simulink model "MIMOOO_FIXED"  (R2022a)
settings: Solver=VariableStepAuto  StartTime=0.0  StopTime=100  RelTol=1e-3
libraries: dspsigops x80, commchan3 x4, commdigbbndpm3 x2, commfilt2 x2, commsink2 x1, simulink x1
(part 4 of 6)

== system MIMOOO_FIXED/Transceiver1/Interpolation 2/E7 ==
  In1 : Inport
  Data Type Conversion1 : DataTypeConversion  OutDataTypeStr=fixdt(1,19,0)  RndMeth=Floor
  Data Type Conversion12 : DataTypeConversion  OutDataTypeStr=fixdt(1,17,0)  RndMeth=Floor
  Data Type Conversion2 : DataTypeConversion  OutDataTypeStr=fixdt(1,18,0)  RndMeth=Floor
  Data Type Conversion3 : DataTypeConversion  OutDataTypeStr=fixdt(1,19,0)  RndMeth=Floor
  Delay6 : Delay  DelayLength=1
  Delay7 : Delay  DelayLength=1
  Gain4 : Gain  Gain=56
  Gain5 : Gain  Gain=336
  Gain6 : Gain  Gain=120
  Sum4 : Sum
  Sum5 : Sum
  Out1 : Outport
  wires:
  Gain4/1 -> Data Type Conversion12/1
  Sum4/1 -> Data Type Conversion3/1
  Delay7/1 -> Sum5/2
  Gain6/1 -> Data Type Conversion2/1
  Delay6/1 -> Sum4/2
  Data Type Conversion12/1 -> Delay6/1
  Gain5/1 -> Data Type Conversion1/1
  Data Type Conversion1/1 -> Sum4/1
  Data Type Conversion2/1 -> Sum5/1
  Data Type Conversion3/1 -> Delay7/1
  In1/1 -> Gain6/1, Gain5/1, Gain4/1
  Sum5/1 -> Out1/1

== system MIMOOO_FIXED/Transceiver5/ADC 1/SigmaDelta ADC ==
  note: c1
  In : Inport
  Discrete Transfer Fcn : DiscreteTransferFcn  Denominator=[1 -1]
  Discrete Transfer Fcn1 : DiscreteTransferFcn  Numerator=[1 0]  Denominator=[1 -1]
  Discrete Transfer Fcn2 : DiscreteTransferFcn  Denominator=[1 -1]
  Discrete Transfer Fcn3 : DiscreteTransferFcn  Numerator=[1 0]  Denominator=[1 -1]
  Discrete Transfer Fcn4 : DiscreteTransferFcn  Denominator=[1 -1]
  Discrete Transfer Fcn5 : DiscreteTransferFcn  Numerator=[1 0]  Denominator=[1 -1]
  Sign : Signum
  Sum : Sum  Inputs=-++  InputSameDT=on  SaturateOnIntegerOverflow=on  OutDataTypeStr=Inherit: Same as first input
  Sum1 : Sum  Inputs=-+  InputSameDT=on  SaturateOnIntegerOverflow=on  OutDataTypeStr=Inherit: Same as first input
  Sum3 : Sum  Inputs=-+  InputSameDT=on  SaturateOnIntegerOverflow=on  OutDataTypeStr=Inherit: Same as first input
  Sum4 : Sum  Inputs=++++++  InputSameDT=on  SaturateOnIntegerOverflow=on  OutDataTypeStr=Inherit: Same as first input
  a : Gain  Gain=-1  SaturateOnIntegerOverflow=on  OutDataTypeStr=Inherit: Same as input  ParamDataTypeStr=Inherit: Same as input
  a1 : Gain  Gain=0.556869897897495  SaturateOnIntegerOverflow=on  OutDataTypeStr=Inherit: Same as input  ParamDataTypeStr=Inherit: Same as input
  a2 : Gain  Gain=-0.556869897925717  SaturateOnIntegerOverflow=on  OutDataTypeStr=Inherit: Same as input  ParamDataTypeStr=Inherit: Same as input
  a3 : Gain  Gain=5.57074843011795e-10  SaturateOnIntegerOverflow=on  OutDataTypeStr=Inherit: Same as input  ParamDataTypeStr=Inherit: Same as input
  a4 : Gain  Gain=-0.239860502762260  SaturateOnIntegerOverflow=on  OutDataTypeStr=Inherit: Same as input  ParamDataTypeStr=Inherit: Same as input
  a5 : Gain  Gain=-0.0411685762497780  SaturateOnIntegerOverflow=on  OutDataTypeStr=Inherit: Same as input  ParamDataTypeStr=Inherit: Same as input
  a6 : Gain  Gain=0.0229325751731016  SaturateOnIntegerOverflow=on  OutDataTypeStr=Inherit: Same as input  ParamDataTypeStr=Inherit: Same as input
  gc1 : Gain  Gain=2.00000000000000  SaturateOnIntegerOverflow=on  OutDataTypeStr=Inherit: Same as input  ParamDataTypeStr=Inherit: Same as input
  gc2 : Gain  Gain=2.07602752770857  SaturateOnIntegerOverflow=on  OutDataTypeStr=Inherit: Same as input  ParamDataTypeStr=Inherit: Same as input
  gc3 : Gain  Gain=1.92397247229143  SaturateOnIntegerOverflow=on  OutDataTypeStr=Inherit: Same as input  ParamDataTypeStr=Inherit: Same as input
  Out : Outport
  wires:
  gc1/1 -> Sum/1
  a5/1 -> Sum4/2
  Discrete Transfer Fcn2/1 -> Discrete Transfer Fcn3/1, a3/1
  Sum4/1 -> Sign/1
  Sum1/1 -> Discrete Transfer Fcn2/1
  Sum/1 -> Discrete Transfer Fcn/1
  a1/1 -> Sum4/6
  gc2/1 -> Sum1/1
  a/1 -> Sum/3
  Discrete Transfer Fcn3/1 -> a4/1, Sum3/2, gc2/1
  Discrete Transfer Fcn5/1 -> a6/1, gc3/1
  Discrete Transfer Fcn1/1 -> a2/1, gc1/1, Sum1/2
  In/1 -> Sum/2
  Sign/1 -> Out/1, a/1
  gc3/1 -> Sum3/1
  a3/1 -> Sum4/4
  a4/1 -> Sum4/3
  a2/1 -> Sum4/5
  Discrete Transfer Fcn/1 -> Discrete Transfer Fcn1/1, a1/1
  Sum3/1 -> Discrete Transfer Fcn4/1
  Discrete Transfer Fcn4/1 -> Discrete Transfer Fcn5/1, a5/1
  a6/1 -> Sum4/1

== system MIMOOO_FIXED/Transceiver5/Interpolation 1/Half_band ==
  Input : Inport
  Add2 : Sum
  Delay11 : Delay  DelayLength=1
  E0(Z) : Subsystem
  E1(Z) : Subsystem
  Upsample 1 : dspsigops/Upsample  N=2  phase=0  RateOptions=Allow multirate processing  ic=0  mode=Unused parameter value
  Upsample 2 : dspsigops/Upsample  N=2  phase=0  RateOptions=Allow multirate processing  ic=0  mode=Unused parameter value
  Out1 : Outport
  wires:
  Upsample 2/1 -> Delay11/1
  Upsample 1/1 -> Add2/1
  E1(Z)/1(Output) -> Upsample 2/1
  Delay11/1 -> Add2/2
  E0(Z)/1(Out1) -> Upsample 1/1
  Add2/1 -> Out1/1
  Input/1 -> E0(Z)/1(Input), E1(Z)/1(Input1)

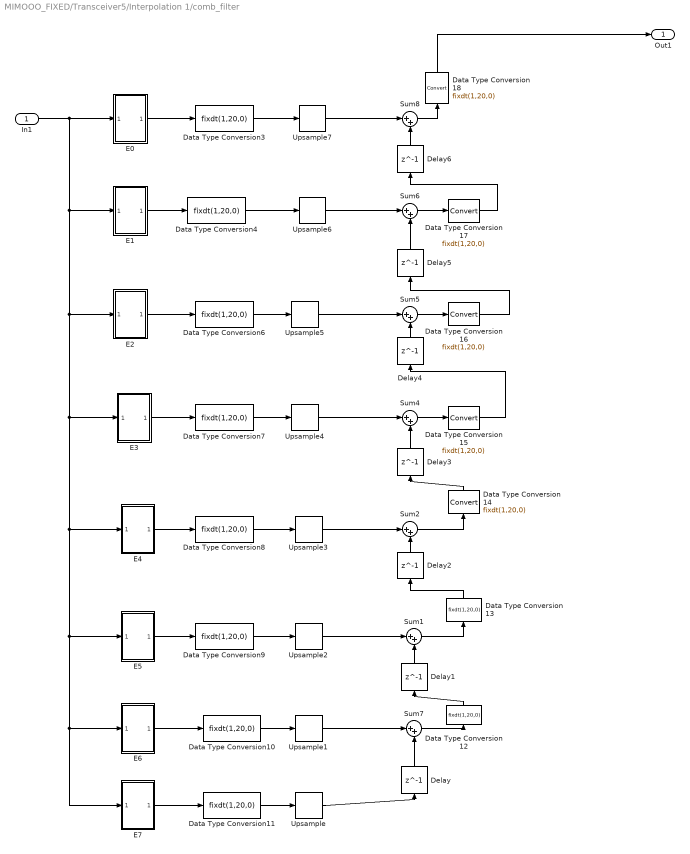
== system MIMOOO_FIXED/Transceiver5/Interpolation 1/comb_filter ==
  In1 : Inport
  Data Type Conversion{3..4,6..18} (15 alike) : DataTypeConversion  OutDataTypeStr=fixdt(1,20,0)  RndMeth=Floor
  Delay{,1..6} (7 alike) : Delay  DelayLength=1
  E0 : Subsystem
  E1 : Subsystem
  E2 : Subsystem
  E3 : Subsystem
  E4 : Subsystem
  E5 : Subsystem
  E6 : Subsystem
  E7 : Subsystem
  Sum{1..2,4..8} (7 alike) : Sum  Inputs=|++
  Upsample{,1..7} (8 alike) : dspsigops/Upsample  N=8  phase=0  RateOptions=Allow multirate processing  ic=0  mode=Unused parameter value
  Out1 : Outport
  wires:
  Upsample7/1 -> Sum8/1
  E4/1(Out1) -> Data Type Conversion8/1
  Data Type Conversion4/1 -> Upsample6/1
  E6/1(Out1) -> Data Type Conversion10/1
  Delay4/1 -> Sum5/2
  Data Type Conversion13/1 -> Delay2/1
  Delay5/1 -> Sum6/2
  Data Type Conversion9/1 -> Upsample2/1
  Sum8/1 -> Data Type Conversion18/1
  Data Type Conversion3/1 -> Upsample7/1
  Sum6/1 -> Data Type Conversion17/1
  Data Type Conversion15/1 -> Delay4/1
  Data Type Conversion14/1 -> Delay3/1
  Data Type Conversion16/1 -> Delay5/1
  E2/1(Out1) -> Data Type Conversion6/1
  In1/1 -> E0/1(In1), E7/1(In1), E6/1(In1), E5/1(In1), E4/1(In1), E3/1(In1), E2/1(In1), E1/1(In1)
  Delay2/1 -> Sum2/2
  Data Type Conversion17/1 -> Delay6/1
  Sum7/1 -> Data Type Conversion12/1
  Data Type Conversion6/1 -> Upsample5/1
  Sum2/1 -> Data Type Conversion14/1
  Data Type Conversion10/1 -> Upsample1/1
  Upsample/1 -> Delay/1
  Upsample6/1 -> Sum6/1
  E5/1(Out1) -> Data Type Conversion9/1
  Data Type Conversion8/1 -> Upsample3/1
  Data Type Conversion7/1 -> Upsample4/1
  Delay1/1 -> Sum1/2
  Sum5/1 -> Data Type Conversion16/1
  Delay/1 -> Sum7/2
  Upsample3/1 -> Sum2/1
  Data Type Conversion11/1 -> Upsample/1
  Upsample4/1 -> Sum4/1
  E7/1(Out1) -> Data Type Conversion11/1
  Sum1/1 -> Data Type Conversion13/1
  Delay3/1 -> Sum4/2
  E3/1(Out1) -> Data Type Conversion7/1
  Data Type Conversion12/1 -> Delay1/1
  Sum4/1 -> Data Type Conversion15/1
  Upsample2/1 -> Sum1/1
  Upsample5/1 -> Sum5/1
  Upsample1/1 -> Sum7/1
  E1/1(Out1) -> Data Type Conversion4/1
  Delay6/1 -> Sum8/2
  Data Type Conversion18/1 -> Out1/1
  E0/1(Out1) -> Data Type Conversion3/1

== system MIMOOO_FIXED/Transceiver5/Interpolation 2/E0 ==
  In1 : Inport
  Data Type Conversion1 : DataTypeConversion  OutDataTypeStr=fixdt(1,19,0)  RndMeth=Floor
  Data Type Conversion2 : DataTypeConversion  OutDataTypeStr=fixdt(1,18,0)  RndMeth=Floor
  Data Type Conversion3 : DataTypeConversion  OutDataTypeStr=fixdt(1,11,0)  RndMeth=Floor
  Data Type Conversion4 : DataTypeConversion  OutDataTypeStr=fixdt(1,20,0)  RndMeth=Floor
  Data Type Conversion5 : DataTypeConversion  OutDataTypeStr=fixdt(1,20,0)  RndMeth=Floor
  Data Type Conversion7 : DataTypeConversion  OutDataTypeStr=fixdt(1,16,0)  RndMeth=Floor
  Delay3 : Delay  DelayLength=1
  Delay4 : Delay  DelayLength=1
  Delay5 : Delay  DelayLength=1
  Gain : Gain  Gain=35
  Gain1 : Gain  Gain=315
  Gain2 : Gain  Gain=161
  Gain3 : Gain
  Sum : Sum
  Sum1 : Sum
  Sum2 : Sum
  Out1 : Outport
  wires:
  Sum1/1 -> Data Type Conversion5/1
  Delay3/1 -> Sum/2
  Delay5/1 -> Sum2/2
  Data Type Conversion7/1 -> Delay3/1
  Gain/1 -> Data Type Conversion7/1
  Gain1/1 -> Data Type Conversion1/1
  Data Type Conversion1/1 -> Sum/1
  Gain2/1 -> Data Type Conversion2/1
  Data Type Conversion3/1 -> Sum2/1
  Gain3/1 -> Data Type Conversion3/1
  Sum/1 -> Data Type Conversion4/1
  Data Type Conversion4/1 -> Delay4/1
  Data Type Conversion2/1 -> Sum1/1
  Delay4/1 -> Sum1/2
  Data Type Conversion5/1 -> Delay5/1
  In1/1 -> Gain2/1, Gain3/1, Gain1/1, Gain/1
  Sum2/1 -> Out1/1

== system MIMOOO_FIXED/Transceiver5/Interpolation 2/E0(Z) ==
  Input : Inport
  Data Type Conversion5 : DataTypeConversion  OutDataTypeStr=fixdt(1,23,0)  RndMeth=Floor
  Delay : Delay  DelayLength=5
  Gain : Gain  Gain=256
  Out1 : Outport
  wires:
  Input/1 -> Gain/1
  Delay/1 -> Out1/1
  Gain/1 -> Data Type Conversion5/1
  Data Type Conversion5/1 -> Delay/1

== system MIMOOO_FIXED/Transceiver5/Interpolation 2/E1 ==
  In1 : Inport
  Data Type Conversion1 : DataTypeConversion  OutDataTypeStr=fixdt(1,19,0)  RndMeth=Floor
  Data Type Conversion2 : DataTypeConversion  OutDataTypeStr=fixdt(1,19,0)  RndMeth=Floor
  Data Type Conversion3 : DataTypeConversion  OutDataTypeStr=fixdt(1,13,0)  RndMeth=Floor
  Data Type Conversion4 : DataTypeConversion  OutDataTypeStr=fixdt(1,19,0)  RndMeth=Floor
  Data Type Conversion5 : DataTypeConversion  OutDataTypeStr=fixdt(1,20,0)  RndMeth=Floor
  Data Type Conversion7 : DataTypeConversion  OutDataTypeStr=fixdt(1,15,0)  RndMeth=Floor
  Delay3 : Delay  DelayLength=1
  Delay4 : Delay  DelayLength=1
  Delay5 : Delay  DelayLength=1
  Gain : Gain  Gain=20
  Gain1 : Gain  Gain=284
  Gain2 : Gain  Gain=204
  Gain3 : Gain  Gain=4
  Sum : Sum
  Sum1 : Sum
  Sum2 : Sum
  Out1 : Outport
  wires:
  Sum/1 -> Data Type Conversion4/1
  Delay3/1 -> Sum/2
  Delay4/1 -> Sum1/2
  Delay5/1 -> Sum2/2
  Gain/1 -> Data Type Conversion7/1
  Data Type Conversion7/1 -> Delay3/1
  Gain1/1 -> Data Type Conversion1/1
  Data Type Conversion1/1 -> Sum/1
  Gain2/1 -> Data Type Conversion2/1
  Data Type Conversion2/1 -> Sum1/1
  Gain3/1 -> Data Type Conversion3/1
  Data Type Conversion3/1 -> Sum2/1
  Data Type Conversion4/1 -> Delay4/1
  Sum1/1 -> Data Type Conversion5/1
  Data Type Conversion5/1 -> Delay5/1
  In1/1 -> Gain2/1, Gain3/1, Gain1/1, Gain/1
  Sum2/1 -> Out1/1

== system MIMOOO_FIXED/Transceiver5/Interpolation 2/E1(Z) ==
  Input1 : Inport
  10-12 : Gain  Gain=158
  2-20 : Gain
  4-18 : Gain  Gain=-4
  6-16 : Gain  Gain=13
  8-14 : Gain  Gain=-40
  Add{7..10,12..16} (9 alike) : Sum
  Data Type Conversion1 : DataTypeConversion  OutDataTypeStr=fixdt(1,15,0)  RndMeth=Floor
  Data Type Conversion{10..14} (5 alike) : DataTypeConversion  OutDataTypeStr=fixdt(1,23,0)  RndMeth=Floor
  Data Type Conversion2 : DataTypeConversion  OutDataTypeStr=fixdt(1,17,0)  RndMeth=Floor
  Data Type Conversion3 : DataTypeConversion  OutDataTypeStr=fixdt(1,19,0)  RndMeth=Floor
  Data Type Conversion4 : DataTypeConversion  OutDataTypeStr=fixdt(1,20,0)  RndMeth=Floor
  Data Type Conversion5 : DataTypeConversion  OutDataTypeStr=fixdt(1,22,0)  RndMeth=Floor
  Data Type Conversion6 : DataTypeConversion  OutDataTypeStr=fixdt(1,17,0)  RndMeth=Floor
  Data Type Conversion7 : DataTypeConversion  OutDataTypeStr=fixdt(1,19,0)  RndMeth=Floor
  Data Type Conversion8 : DataTypeConversion  OutDataTypeStr=fixdt(1,20,0)  RndMeth=Floor
  Data Type Conversion9 : DataTypeConversion  OutDataTypeStr=fixdt(1,22,0)  RndMeth=Floor
  Delay{21,23,25,27,29,31,33,35,37} (9 alike) : Delay  DelayLength=1
  Output : Outport
  wires:
  8-14/1 -> Data Type Conversion4/1
  Delay29/1 -> Add12/2  "x[n-11]"
  Add14/1 -> Data Type Conversion12/1
  Input1/1 -> 2-20/1, 10-12/1, 8-14/1, 6-16/1, 4-18/1
  4-18/1 -> Data Type Conversion2/1
  Delay33/1 -> Add14/2
  Add12/1 -> Data Type Conversion10/1
  10-12/1 -> Data Type Conversion5/1
  Delay37/1 -> Add16/2  "x[n-19]"
  6-16/1 -> Data Type Conversion3/1
  Delay25/1 -> Add9/2  "x[n-7]"
  Add7/1 -> Data Type Conversion6/1
  Add15/1 -> Data Type Conversion13/1
  Delay23/1 -> Add8/2  "x[n-5]"
  Delay27/1 -> Add10/2  "x[n-9]"
  Delay31/1 -> Add13/2  "x[n-13]"
  Delay35/1 -> Add15/2  "x[n-17]"
  Delay21/1 -> Add7/2  "x[n-3]"
  2-20/1 -> Data Type Conversion1/1
  Add13/1 -> Data Type Conversion11/1
  Add10/1 -> Data Type Conversion9/1
  Data Type Conversion1/1 -> Delay21/1, Add16/1
  Data Type Conversion2/1 -> Add7/1, Add15/1
  Data Type Conversion3/1 -> Add8/1, Add14/1
  Data Type Conversion4/1 -> Add9/1, Add13/1
  Data Type Conversion5/1 -> Add10/1, Add12/1
  Data Type Conversion6/1 -> Delay23/1
  Add8/1 -> Data Type Conversion7/1
  Data Type Conversion7/1 -> Delay25/1
  Add9/1 -> Data Type Conversion8/1
  Data Type Conversion8/1 -> Delay27/1
  Data Type Conversion9/1 -> Delay29/1
  Data Type Conversion10/1 -> Delay31/1
  Data Type Conversion11/1 -> Delay33/1
  Data Type Conversion12/1 -> Delay35/1
  Data Type Conversion13/1 -> Delay37/1
  Add16/1 -> Data Type Conversion14/1
  Data Type Conversion14/1 -> Output/1

== system MIMOOO_FIXED/Transceiver5/Interpolation 2/E2 ==
  In1 : Inport
  Data Type Conversion : DataTypeConversion  OutDataTypeStr=fixdt(1,14,0)  SaturateOnIntegerOverflow=off  RndMeth=Floor
  Data Type Conversion1 : DataTypeConversion  OutDataTypeStr=fixdt(1,19,0)  SaturateOnIntegerOverflow=off  RndMeth=Floor
  Data Type Conversion2 : DataTypeConversion  OutDataTypeStr=fixdt(1,19,0)  SaturateOnIntegerOverflow=off  RndMeth=Floor
  Data Type Conversion3 : DataTypeConversion  OutDataTypeStr=fixdt(1,20,0)  SaturateOnIntegerOverflow=off  RndMeth=Floor
  Delay3 : Delay  DelayLength=1
  Delay4 : Delay  DelayLength=1
  Delay5 : Delay  DelayLength=1
  Gain : Gain  Gain=10
  Gain1 : Gain  Gain=246
  Sum : Sum
  Sum1 : Sum
  Sum2 : Sum
  Out1 : Outport
  wires:
  Sum1/1 -> Data Type Conversion3/1
  Delay3/1 -> Sum/2
  Delay4/1 -> Sum1/2
  Delay5/1 -> Sum2/2
  Data Type Conversion/1 -> Delay3/1, Sum2/1
  Gain/1 -> Data Type Conversion/1
  Gain1/1 -> Data Type Conversion1/1
  Data Type Conversion1/1 -> Sum1/1, Sum/1
  Data Type Conversion2/1 -> Delay4/1
  Sum/1 -> Data Type Conversion2/1
  Data Type Conversion3/1 -> Delay5/1
  In1/1 -> Gain1/1, Gain/1
  Sum2/1 -> Out1/1

== system MIMOOO_FIXED/Transceiver5/Interpolation 2/E3 ==
  In1 : Inport
  Data Type Conversion : DataTypeConversion  OutDataTypeStr=fixdt(1,13,0)  SaturateOnIntegerOverflow=off  RndMeth=Floor
  Data Type Conversion1 : DataTypeConversion  OutDataTypeStr=fixdt(1,19,0)  SaturateOnIntegerOverflow=off  RndMeth=Floor
  Data Type Conversion2 : DataTypeConversion  OutDataTypeStr=fixdt(1,19,0)  SaturateOnIntegerOverflow=off  RndMeth=Floor
  Data Type Conversion3 : DataTypeConversion  OutDataTypeStr=fixdt(1,15,0)  SaturateOnIntegerOverflow=off  RndMeth=Floor
  Data Type Conversion4 : DataTypeConversion  OutDataTypeStr=fixdt(1,19,0)  SaturateOnIntegerOverflow=off  RndMeth=Floor
  Data Type Conversion5 : DataTypeConversion  OutDataTypeStr=fixdt(1,20,0)  SaturateOnIntegerOverflow=off  RndMeth=Floor
  Delay3 : Delay  DelayLength=1
  Delay4 : Delay  DelayLength=1
  Delay5 : Delay  DelayLength=1
  Gain : Gain  Gain=4
  Gain1 : Gain  Gain=204
  Gain2 : Gain  Gain=284
  Gain3 : Gain  Gain=20
  Sum : Sum
  Sum1 : Sum
  Sum2 : Sum
  Out1 : Outport
  wires:
  Delay3/1 -> Sum/2
  Delay4/1 -> Sum1/2
  Delay5/1 -> Sum2/2
  Gain/1 -> Data Type Conversion/1
  Data Type Conversion/1 -> Delay3/1
  Gain1/1 -> Data Type Conversion1/1
  Data Type Conversion1/1 -> Sum/1
  Gain2/1 -> Data Type Conversion2/1
  Data Type Conversion2/1 -> Sum1/1
  Gain3/1 -> Data Type Conversion3/1
  Data Type Conversion3/1 -> Sum2/1
  Sum/1 -> Data Type Conversion4/1
  Data Type Conversion4/1 -> Delay4/1
  Sum1/1 -> Data Type Conversion5/1
  Data Type Conversion5/1 -> Delay5/1
  Sum2/1 -> Out1/1
  In1/1 -> Gain3/1, Gain2/1, Gain1/1, Gain/1

== system MIMOOO_FIXED/Transceiver5/Interpolation 2/E4 ==
  In1 : Inport
  Data Type Conversion1 : DataTypeConversion  OutDataTypeStr=fixdt(1,18,0)  RndMeth=Floor
  Data Type Conversion12 : DataTypeConversion  OutDataTypeStr=fixdt(1,11,0)  RndMeth=Floor
  Data Type Conversion2 : DataTypeConversion  OutDataTypeStr=fixdt(1,19,0)  RndMeth=Floor
  Data Type Conversion3 : DataTypeConversion  OutDataTypeStr=fixdt(1,16,0)  RndMeth=Floor
  Data Type Conversion4 : DataTypeConversion  OutDataTypeStr=fixdt(1,18,0)  RndMeth=Floor
  Data Type Conversion5 : DataTypeConversion  OutDataTypeStr=fixdt(1,19,0)  RndMeth=Floor
  Delay3 : Delay  DelayLength=1
  Delay4 : Delay  DelayLength=1
  Delay5 : Delay  DelayLength=1
  Gain : Gain
  Gain1 : Gain  Gain=161
  Gain2 : Gain  Gain=315
  Gain3 : Gain  Gain=35
  Sum : Sum
  Sum1 : Sum
  Sum2 : Sum
  Out1 : Outport
  wires:
  Sum1/1 -> Data Type Conversion5/1
  Sum/1 -> Data Type Conversion4/1
  Gain1/1 -> Data Type Conversion1/1
  Delay3/1 -> Sum/2
  Delay4/1 -> Sum1/2
  Gain3/1 -> Data Type Conversion3/1
  Delay5/1 -> Sum2/2
  Gain/1 -> Data Type Conversion12/1
  Data Type Conversion12/1 -> Delay3/1
  Data Type Conversion1/1 -> Sum/1
  Gain2/1 -> Data Type Conversion2/1
  Data Type Conversion2/1 -> Sum1/1
  Data Type Conversion3/1 -> Sum2/1
  Data Type Conversion4/1 -> Delay4/1
  Data Type Conversion5/1 -> Delay5/1
  In1/1 -> Gain2/1, Gain3/1, Gain1/1, Gain/1
  Sum2/1 -> Out1/1

== system MIMOOO_FIXED/Transceiver5/Interpolation 2/E5 ==
  In1 : Inport
  Data Type Conversion1 : DataTypeConversion  OutDataTypeStr=fixdt(1,19,0)  RndMeth=Floor
  Data Type Conversion12 : DataTypeConversion  OutDataTypeStr=fixdt(1,18,0)  RndMeth=Floor
  Data Type Conversion2 : DataTypeConversion  OutDataTypeStr=fixdt(1,17,0)  RndMeth=Floor
  Data Type Conversion3 : DataTypeConversion  OutDataTypeStr=fixdt(1,19,0)  RndMeth=Floor
  Delay6 : Delay  DelayLength=1
  Delay7 : Delay  DelayLength=1
  Gain4 : Gain  Gain=120
  Gain5 : Gain  Gain=336
  Gain6 : Gain  Gain=56
  Sum4 : Sum
  Sum5 : Sum
  Out1 : Outport
  wires:
  Gain4/1 -> Data Type Conversion12/1
  Sum4/1 -> Data Type Conversion3/1
  Delay7/1 -> Sum5/2
  Gain6/1 -> Data Type Conversion2/1
  Delay6/1 -> Sum4/2
  Data Type Conversion12/1 -> Delay6/1
  Gain5/1 -> Data Type Conversion1/1
  Data Type Conversion1/1 -> Sum4/1
  Data Type Conversion2/1 -> Sum5/1
  Data Type Conversion3/1 -> Delay7/1
  In1/1 -> Gain6/1, Gain5/1, Gain4/1
  Sum5/1 -> Out1/1

== system MIMOOO_FIXED/Transceiver5/Interpolation 2/E6 ==
  In1 : Inport
  Data Type Conversion1 : DataTypeConversion  OutDataTypeStr=fixdt(1,20,0)  RndMeth=Floor
  Data Type Conversion2 : DataTypeConversion  OutDataTypeStr=fixdt(1,20,0)  RndMeth=Floor
  Data Type Conversion3 : DataTypeConversion  OutDataTypeStr=fixdt(1,17,0)  RndMeth=Floor
  Delay6 : Delay  DelayLength=1
  Delay7 : Delay  DelayLength=1
  Gain4 : Gain  Gain=84
  Gain5 : Gain  Gain=344
  Sum4 : Sum
  Sum5 : Sum
  Out1 : Outport
  wires:
  Delay7/1 -> Sum5/2
  Gain4/1 -> Data Type Conversion3/1
  Gain5/1 -> Data Type Conversion1/1
  Delay6/1 -> Sum4/2
  Data Type Conversion3/1 -> Sum5/1, Delay6/1
  Data Type Conversion1/1 -> Sum4/1
  Sum4/1 -> Data Type Conversion2/1
  Data Type Conversion2/1 -> Delay7/1
  In1/1 -> Gain5/1, Gain4/1
  Sum5/1 -> Out1/1

== system MIMOOO_FIXED/Transceiver5/Interpolation 2/E7 ==
  In1 : Inport
  Data Type Conversion1 : DataTypeConversion  OutDataTypeStr=fixdt(1,19,0)  RndMeth=Floor
  Data Type Conversion12 : DataTypeConversion  OutDataTypeStr=fixdt(1,17,0)  RndMeth=Floor
  Data Type Conversion2 : DataTypeConversion  OutDataTypeStr=fixdt(1,18,0)  RndMeth=Floor
  Data Type Conversion3 : DataTypeConversion  OutDataTypeStr=fixdt(1,19,0)  RndMeth=Floor
  Delay6 : Delay  DelayLength=1
  Delay7 : Delay  DelayLength=1
  Gain4 : Gain  Gain=56
  Gain5 : Gain  Gain=336
  Gain6 : Gain  Gain=120
  Sum4 : Sum
  Sum5 : Sum
  Out1 : Outport
  wires:
  Gain4/1 -> Data Type Conversion12/1
  Sum4/1 -> Data Type Conversion3/1
  Delay7/1 -> Sum5/2
  Gain6/1 -> Data Type Conversion2/1
  Delay6/1 -> Sum4/2
  Data Type Conversion12/1 -> Delay6/1
  Gain5/1 -> Data Type Conversion1/1
  Data Type Conversion1/1 -> Sum4/1
  Data Type Conversion2/1 -> Sum5/1
  Data Type Conversion3/1 -> Delay7/1
  In1/1 -> Gain6/1, Gain5/1, Gain4/1
  Sum5/1 -> Out1/1

== system MIMOOO_FIXED/Transceiver6/ADC 1/SigmaDelta ADC ==
  note: c1
  In : Inport
  Discrete Transfer Fcn : DiscreteTransferFcn  Denominator=[1 -1]
  Discrete Transfer Fcn1 : DiscreteTransferFcn  Numerator=[1 0]  Denominator=[1 -1]
  Discrete Transfer Fcn2 : DiscreteTransferFcn  Denominator=[1 -1]
  Discrete Transfer Fcn3 : DiscreteTransferFcn  Numerator=[1 0]  Denominator=[1 -1]
  Discrete Transfer Fcn4 : DiscreteTransferFcn  Denominator=[1 -1]
  Discrete Transfer Fcn5 : DiscreteTransferFcn  Numerator=[1 0]  Denominator=[1 -1]
  Sign : Signum
  Sum : Sum  Inputs=-++  InputSameDT=on  SaturateOnIntegerOverflow=on  OutDataTypeStr=Inherit: Same as first input
  Sum1 : Sum  Inputs=-+  InputSameDT=on  SaturateOnIntegerOverflow=on  OutDataTypeStr=Inherit: Same as first input
  Sum3 : Sum  Inputs=-+  InputSameDT=on  SaturateOnIntegerOverflow=on  OutDataTypeStr=Inherit: Same as first input
  Sum4 : Sum  Inputs=++++++  InputSameDT=on  SaturateOnIntegerOverflow=on  OutDataTypeStr=Inherit: Same as first input
  a : Gain  Gain=-1  SaturateOnIntegerOverflow=on  OutDataTypeStr=Inherit: Same as input  ParamDataTypeStr=Inherit: Same as input
  a1 : Gain  Gain=0.556869897897495  SaturateOnIntegerOverflow=on  OutDataTypeStr=Inherit: Same as input  ParamDataTypeStr=Inherit: Same as input
  a2 : Gain  Gain=-0.556869897925717  SaturateOnIntegerOverflow=on  OutDataTypeStr=Inherit: Same as input  ParamDataTypeStr=Inherit: Same as input
  a3 : Gain  Gain=5.57074843011795e-10  SaturateOnIntegerOverflow=on  OutDataTypeStr=Inherit: Same as input  ParamDataTypeStr=Inherit: Same as input
  a4 : Gain  Gain=-0.239860502762260  SaturateOnIntegerOverflow=on  OutDataTypeStr=Inherit: Same as input  ParamDataTypeStr=Inherit: Same as input
  a5 : Gain  Gain=-0.0411685762497780  SaturateOnIntegerOverflow=on  OutDataTypeStr=Inherit: Same as input  ParamDataTypeStr=Inherit: Same as input
  a6 : Gain  Gain=0.0229325751731016  SaturateOnIntegerOverflow=on  OutDataTypeStr=Inherit: Same as input  ParamDataTypeStr=Inherit: Same as input
  gc1 : Gain  Gain=2.00000000000000  SaturateOnIntegerOverflow=on  OutDataTypeStr=Inherit: Same as input  ParamDataTypeStr=Inherit: Same as input
  gc2 : Gain  Gain=2.07602752770857  SaturateOnIntegerOverflow=on  OutDataTypeStr=Inherit: Same as input  ParamDataTypeStr=Inherit: Same as input
  gc3 : Gain  Gain=1.92397247229143  SaturateOnIntegerOverflow=on  OutDataTypeStr=Inherit: Same as input  ParamDataTypeStr=Inherit: Same as input
  Out : Outport
  wires:
  gc1/1 -> Sum/1
  a5/1 -> Sum4/2
  Discrete Transfer Fcn2/1 -> Discrete Transfer Fcn3/1, a3/1
  Sum4/1 -> Sign/1
  Sum1/1 -> Discrete Transfer Fcn2/1
  Sum/1 -> Discrete Transfer Fcn/1
  a1/1 -> Sum4/6
  gc2/1 -> Sum1/1
  a/1 -> Sum/3
  Discrete Transfer Fcn3/1 -> a4/1, Sum3/2, gc2/1
  Discrete Transfer Fcn5/1 -> a6/1, gc3/1
  Discrete Transfer Fcn1/1 -> a2/1, gc1/1, Sum1/2
  In/1 -> Sum/2
  Sign/1 -> Out/1, a/1
  gc3/1 -> Sum3/1
  a3/1 -> Sum4/4
  a4/1 -> Sum4/3
  a2/1 -> Sum4/5
  Discrete Transfer Fcn/1 -> Discrete Transfer Fcn1/1, a1/1
  Sum3/1 -> Discrete Transfer Fcn4/1
  Discrete Transfer Fcn4/1 -> Discrete Transfer Fcn5/1, a5/1
  a6/1 -> Sum4/1

== system MIMOOO_FIXED/Transceiver6/Interpolation 1/Half_band ==
  Input : Inport
  Add2 : Sum
  Delay11 : Delay  DelayLength=1
  E0(Z) : Subsystem
  E1(Z) : Subsystem
  Upsample 1 : dspsigops/Upsample  N=2  phase=0  RateOptions=Allow multirate processing  ic=0  mode=Unused parameter value
  Upsample 2 : dspsigops/Upsample  N=2  phase=0  RateOptions=Allow multirate processing  ic=0  mode=Unused parameter value
  Out1 : Outport
  wires:
  Upsample 2/1 -> Delay11/1
  Upsample 1/1 -> Add2/1
  E1(Z)/1(Output) -> Upsample 2/1
  Delay11/1 -> Add2/2
  E0(Z)/1(Out1) -> Upsample 1/1
  Add2/1 -> Out1/1
  Input/1 -> E0(Z)/1(Input), E1(Z)/1(Input1)

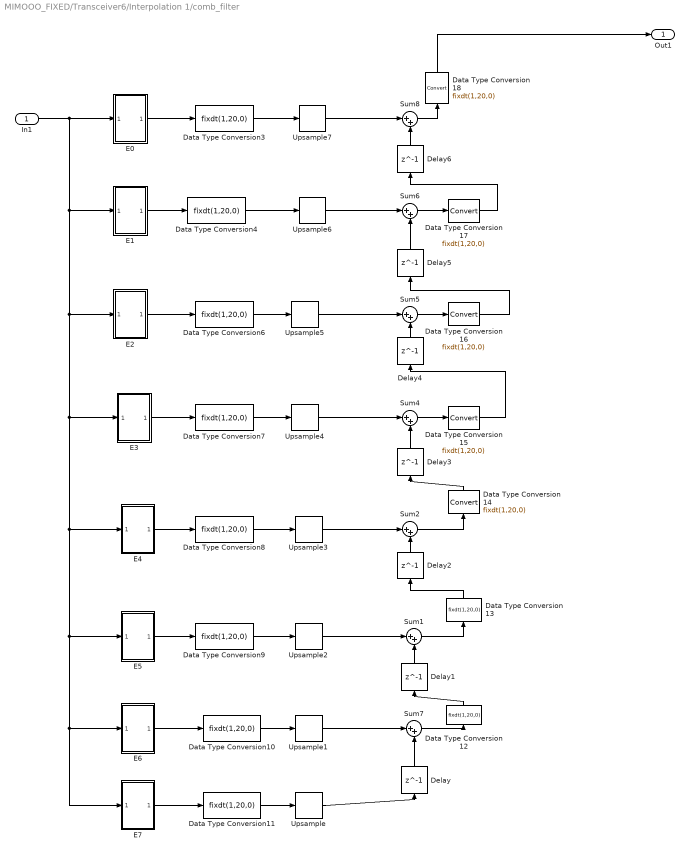
== system MIMOOO_FIXED/Transceiver6/Interpolation 1/comb_filter ==
  In1 : Inport
  Data Type Conversion{3..4,6..18} (15 alike) : DataTypeConversion  OutDataTypeStr=fixdt(1,20,0)  RndMeth=Floor
  Delay{,1..6} (7 alike) : Delay  DelayLength=1
  E0 : Subsystem
  E1 : Subsystem
  E2 : Subsystem
  E3 : Subsystem
  E4 : Subsystem
  E5 : Subsystem
  E6 : Subsystem
  E7 : Subsystem
  Sum{1..2,4..8} (7 alike) : Sum  Inputs=|++
  Upsample{,1..7} (8 alike) : dspsigops/Upsample  N=8  phase=0  RateOptions=Allow multirate processing  ic=0  mode=Unused parameter value
  Out1 : Outport
  wires:
  Upsample7/1 -> Sum8/1
  E4/1(Out1) -> Data Type Conversion8/1
  Data Type Conversion4/1 -> Upsample6/1
  E6/1(Out1) -> Data Type Conversion10/1
  Delay4/1 -> Sum5/2
  Data Type Conversion13/1 -> Delay2/1
  Delay5/1 -> Sum6/2
  Data Type Conversion9/1 -> Upsample2/1
  Sum8/1 -> Data Type Conversion18/1
  Data Type Conversion3/1 -> Upsample7/1
  Sum6/1 -> Data Type Conversion17/1
  Data Type Conversion15/1 -> Delay4/1
  Data Type Conversion14/1 -> Delay3/1
  Data Type Conversion16/1 -> Delay5/1
  E2/1(Out1) -> Data Type Conversion6/1
  In1/1 -> E0/1(In1), E7/1(In1), E6/1(In1), E5/1(In1), E4/1(In1), E3/1(In1), E2/1(In1), E1/1(In1)
  Delay2/1 -> Sum2/2
  Data Type Conversion17/1 -> Delay6/1
  Sum7/1 -> Data Type Conversion12/1
  Data Type Conversion6/1 -> Upsample5/1
  Sum2/1 -> Data Type Conversion14/1
  Data Type Conversion10/1 -> Upsample1/1
  Upsample/1 -> Delay/1
  Upsample6/1 -> Sum6/1
  E5/1(Out1) -> Data Type Conversion9/1
  Data Type Conversion8/1 -> Upsample3/1
  Data Type Conversion7/1 -> Upsample4/1
  Delay1/1 -> Sum1/2
  Sum5/1 -> Data Type Conversion16/1
  Delay/1 -> Sum7/2
  Upsample3/1 -> Sum2/1
  Data Type Conversion11/1 -> Upsample/1
  Upsample4/1 -> Sum4/1
  E7/1(Out1) -> Data Type Conversion11/1
  Sum1/1 -> Data Type Conversion13/1
  Delay3/1 -> Sum4/2
  E3/1(Out1) -> Data Type Conversion7/1
  Data Type Conversion12/1 -> Delay1/1
  Sum4/1 -> Data Type Conversion15/1
  Upsample2/1 -> Sum1/1
  Upsample5/1 -> Sum5/1
  Upsample1/1 -> Sum7/1
  E1/1(Out1) -> Data Type Conversion4/1
  Delay6/1 -> Sum8/2
  Data Type Conversion18/1 -> Out1/1
  E0/1(Out1) -> Data Type Conversion3/1

== system MIMOOO_FIXED/Transceiver6/Interpolation 2/E0 ==
  In1 : Inport
  Data Type Conversion1 : DataTypeConversion  OutDataTypeStr=fixdt(1,19,0)  RndMeth=Floor
  Data Type Conversion2 : DataTypeConversion  OutDataTypeStr=fixdt(1,18,0)  RndMeth=Floor
  Data Type Conversion3 : DataTypeConversion  OutDataTypeStr=fixdt(1,11,0)  RndMeth=Floor
  Data Type Conversion4 : DataTypeConversion  OutDataTypeStr=fixdt(1,20,0)  RndMeth=Floor
  Data Type Conversion5 : DataTypeConversion  OutDataTypeStr=fixdt(1,20,0)  RndMeth=Floor
  Data Type Conversion7 : DataTypeConversion  OutDataTypeStr=fixdt(1,16,0)  RndMeth=Floor
  Delay3 : Delay  DelayLength=1
  Delay4 : Delay  DelayLength=1
  Delay5 : Delay  DelayLength=1
  Gain : Gain  Gain=35
  Gain1 : Gain  Gain=315
  Gain2 : Gain  Gain=161
  Gain3 : Gain
  Sum : Sum
  Sum1 : Sum
  Sum2 : Sum
  Out1 : Outport
  wires:
  Sum1/1 -> Data Type Conversion5/1
  Delay3/1 -> Sum/2
  Delay5/1 -> Sum2/2
  Data Type Conversion7/1 -> Delay3/1
  Gain/1 -> Data Type Conversion7/1
  Gain1/1 -> Data Type Conversion1/1
  Data Type Conversion1/1 -> Sum/1
  Gain2/1 -> Data Type Conversion2/1
  Data Type Conversion3/1 -> Sum2/1
  Gain3/1 -> Data Type Conversion3/1
  Sum/1 -> Data Type Conversion4/1
  Data Type Conversion4/1 -> Delay4/1
  Data Type Conversion2/1 -> Sum1/1
  Delay4/1 -> Sum1/2
  Data Type Conversion5/1 -> Delay5/1
  In1/1 -> Gain2/1, Gain3/1, Gain1/1, Gain/1
  Sum2/1 -> Out1/1

== system MIMOOO_FIXED/Transceiver6/Interpolation 2/E0(Z) ==
  Input : Inport
  Data Type Conversion5 : DataTypeConversion  OutDataTypeStr=fixdt(1,23,0)  RndMeth=Floor
  Delay : Delay  DelayLength=5
  Gain : Gain  Gain=256
  Out1 : Outport
  wires:
  Input/1 -> Gain/1
  Delay/1 -> Out1/1
  Gain/1 -> Data Type Conversion5/1
  Data Type Conversion5/1 -> Delay/1

== system MIMOOO_FIXED/Transceiver6/Interpolation 2/E1 ==
  In1 : Inport
  Data Type Conversion1 : DataTypeConversion  OutDataTypeStr=fixdt(1,19,0)  RndMeth=Floor
  Data Type Conversion2 : DataTypeConversion  OutDataTypeStr=fixdt(1,19,0)  RndMeth=Floor
  Data Type Conversion3 : DataTypeConversion  OutDataTypeStr=fixdt(1,13,0)  RndMeth=Floor
  Data Type Conversion4 : DataTypeConversion  OutDataTypeStr=fixdt(1,19,0)  RndMeth=Floor
  Data Type Conversion5 : DataTypeConversion  OutDataTypeStr=fixdt(1,20,0)  RndMeth=Floor
  Data Type Conversion7 : DataTypeConversion  OutDataTypeStr=fixdt(1,15,0)  RndMeth=Floor
  Delay3 : Delay  DelayLength=1
  Delay4 : Delay  DelayLength=1
  Delay5 : Delay  DelayLength=1
  Gain : Gain  Gain=20
  Gain1 : Gain  Gain=284
  Gain2 : Gain  Gain=204
  Gain3 : Gain  Gain=4
  Sum : Sum
  Sum1 : Sum
  Sum2 : Sum
  Out1 : Outport
  wires:
  Sum/1 -> Data Type Conversion4/1
  Delay3/1 -> Sum/2
  Delay4/1 -> Sum1/2
  Delay5/1 -> Sum2/2
  Gain/1 -> Data Type Conversion7/1
  Data Type Conversion7/1 -> Delay3/1
  Gain1/1 -> Data Type Conversion1/1
  Data Type Conversion1/1 -> Sum/1
  Gain2/1 -> Data Type Conversion2/1
  Data Type Conversion2/1 -> Sum1/1
  Gain3/1 -> Data Type Conversion3/1
  Data Type Conversion3/1 -> Sum2/1
  Data Type Conversion4/1 -> Delay4/1
  Sum1/1 -> Data Type Conversion5/1
  Data Type Conversion5/1 -> Delay5/1
  In1/1 -> Gain2/1, Gain3/1, Gain1/1, Gain/1
  Sum2/1 -> Out1/1

== system MIMOOO_FIXED/Transceiver6/Interpolation 2/E1(Z) ==
  Input1 : Inport
  10-12 : Gain  Gain=158
  2-20 : Gain
  4-18 : Gain  Gain=-4
  6-16 : Gain  Gain=13
  8-14 : Gain  Gain=-40
  Add{7..10,12..16} (9 alike) : Sum
  Data Type Conversion1 : DataTypeConversion  OutDataTypeStr=fixdt(1,15,0)  RndMeth=Floor
  Data Type Conversion{10..14} (5 alike) : DataTypeConversion  OutDataTypeStr=fixdt(1,23,0)  RndMeth=Floor
  Data Type Conversion2 : DataTypeConversion  OutDataTypeStr=fixdt(1,17,0)  RndMeth=Floor
  Data Type Conversion3 : DataTypeConversion  OutDataTypeStr=fixdt(1,19,0)  RndMeth=Floor
  Data Type Conversion4 : DataTypeConversion  OutDataTypeStr=fixdt(1,20,0)  RndMeth=Floor
  Data Type Conversion5 : DataTypeConversion  OutDataTypeStr=fixdt(1,22,0)  RndMeth=Floor
  Data Type Conversion6 : DataTypeConversion  OutDataTypeStr=fixdt(1,17,0)  RndMeth=Floor
  Data Type Conversion7 : DataTypeConversion  OutDataTypeStr=fixdt(1,19,0)  RndMeth=Floor
  Data Type Conversion8 : DataTypeConversion  OutDataTypeStr=fixdt(1,20,0)  RndMeth=Floor
  Data Type Conversion9 : DataTypeConversion  OutDataTypeStr=fixdt(1,22,0)  RndMeth=Floor
  Delay{21,23,25,27,29,31,33,35,37} (9 alike) : Delay  DelayLength=1
  Output : Outport
  wires:
  8-14/1 -> Data Type Conversion4/1
  Delay29/1 -> Add12/2  "x[n-11]"
  Add14/1 -> Data Type Conversion12/1
  Input1/1 -> 2-20/1, 10-12/1, 8-14/1, 6-16/1, 4-18/1
  4-18/1 -> Data Type Conversion2/1
  Delay33/1 -> Add14/2
  Add12/1 -> Data Type Conversion10/1
  10-12/1 -> Data Type Conversion5/1
  Delay37/1 -> Add16/2  "x[n-19]"
  6-16/1 -> Data Type Conversion3/1
  Delay25/1 -> Add9/2  "x[n-7]"
  Add7/1 -> Data Type Conversion6/1
  Add15/1 -> Data Type Conversion13/1
  Delay23/1 -> Add8/2  "x[n-5]"
  Delay27/1 -> Add10/2  "x[n-9]"
  Delay31/1 -> Add13/2  "x[n-13]"
  Delay35/1 -> Add15/2  "x[n-17]"
  Delay21/1 -> Add7/2  "x[n-3]"
  2-20/1 -> Data Type Conversion1/1
  Add13/1 -> Data Type Conversion11/1
  Add10/1 -> Data Type Conversion9/1
  Data Type Conversion1/1 -> Delay21/1, Add16/1
  Data Type Conversion2/1 -> Add7/1, Add15/1
  Data Type Conversion3/1 -> Add8/1, Add14/1
  Data Type Conversion4/1 -> Add9/1, Add13/1
  Data Type Conversion5/1 -> Add10/1, Add12/1
  Data Type Conversion6/1 -> Delay23/1
  Add8/1 -> Data Type Conversion7/1
  Data Type Conversion7/1 -> Delay25/1
  Add9/1 -> Data Type Conversion8/1
  Data Type Conversion8/1 -> Delay27/1
  Data Type Conversion9/1 -> Delay29/1
  Data Type Conversion10/1 -> Delay31/1
  Data Type Conversion11/1 -> Delay33/1
  Data Type Conversion12/1 -> Delay35/1
  Data Type Conversion13/1 -> Delay37/1
  Add16/1 -> Data Type Conversion14/1
  Data Type Conversion14/1 -> Output/1

== system MIMOOO_FIXED/Transceiver6/Interpolation 2/E2 ==
  In1 : Inport
  Data Type Conversion : DataTypeConversion  OutDataTypeStr=fixdt(1,14,0)  SaturateOnIntegerOverflow=off  RndMeth=Floor
  Data Type Conversion1 : DataTypeConversion  OutDataTypeStr=fixdt(1,19,0)  SaturateOnIntegerOverflow=off  RndMeth=Floor
  Data Type Conversion2 : DataTypeConversion  OutDataTypeStr=fixdt(1,19,0)  SaturateOnIntegerOverflow=off  RndMeth=Floor
  Data Type Conversion3 : DataTypeConversion  OutDataTypeStr=fixdt(1,20,0)  SaturateOnIntegerOverflow=off  RndMeth=Floor
  Delay3 : Delay  DelayLength=1
  Delay4 : Delay  DelayLength=1
  Delay5 : Delay  DelayLength=1
  Gain : Gain  Gain=10
  Gain1 : Gain  Gain=246
  Sum : Sum
  Sum1 : Sum
  Sum2 : Sum
  Out1 : Outport
  wires:
  Sum1/1 -> Data Type Conversion3/1
  Delay3/1 -> Sum/2
  Delay4/1 -> Sum1/2
  Delay5/1 -> Sum2/2
  Data Type Conversion/1 -> Delay3/1, Sum2/1
  Gain/1 -> Data Type Conversion/1
  Gain1/1 -> Data Type Conversion1/1
  Data Type Conversion1/1 -> Sum1/1, Sum/1
  Data Type Conversion2/1 -> Delay4/1
  Sum/1 -> Data Type Conversion2/1
  Data Type Conversion3/1 -> Delay5/1
  In1/1 -> Gain1/1, Gain/1
  Sum2/1 -> Out1/1

== system MIMOOO_FIXED/Transceiver6/Interpolation 2/E3 ==
  In1 : Inport
  Data Type Conversion : DataTypeConversion  OutDataTypeStr=fixdt(1,13,0)  SaturateOnIntegerOverflow=off  RndMeth=Floor
  Data Type Conversion1 : DataTypeConversion  OutDataTypeStr=fixdt(1,19,0)  SaturateOnIntegerOverflow=off  RndMeth=Floor
  Data Type Conversion2 : DataTypeConversion  OutDataTypeStr=fixdt(1,19,0)  SaturateOnIntegerOverflow=off  RndMeth=Floor
  Data Type Conversion3 : DataTypeConversion  OutDataTypeStr=fixdt(1,15,0)  SaturateOnIntegerOverflow=off  RndMeth=Floor
  Data Type Conversion4 : DataTypeConversion  OutDataTypeStr=fixdt(1,19,0)  SaturateOnIntegerOverflow=off  RndMeth=Floor
  Data Type Conversion5 : DataTypeConversion  OutDataTypeStr=fixdt(1,20,0)  SaturateOnIntegerOverflow=off  RndMeth=Floor
  Delay3 : Delay  DelayLength=1
  Delay4 : Delay  DelayLength=1
  Delay5 : Delay  DelayLength=1
  Gain : Gain  Gain=4
  Gain1 : Gain  Gain=204
  Gain2 : Gain  Gain=284
  Gain3 : Gain  Gain=20
  Sum : Sum
  Sum1 : Sum
  Sum2 : Sum
  Out1 : Outport
  wires:
  Delay3/1 -> Sum/2
  Delay4/1 -> Sum1/2
  Delay5/1 -> Sum2/2
  Gain/1 -> Data Type Conversion/1
  Data Type Conversion/1 -> Delay3/1
  Gain1/1 -> Data Type Conversion1/1
  Data Type Conversion1/1 -> Sum/1
  Gain2/1 -> Data Type Conversion2/1
  Data Type Conversion2/1 -> Sum1/1
  Gain3/1 -> Data Type Conversion3/1
  Data Type Conversion3/1 -> Sum2/1
  Sum/1 -> Data Type Conversion4/1
  Data Type Conversion4/1 -> Delay4/1
  Sum1/1 -> Data Type Conversion5/1
  Data Type Conversion5/1 -> Delay5/1
  Sum2/1 -> Out1/1
  In1/1 -> Gain3/1, Gain2/1, Gain1/1, Gain/1

== system MIMOOO_FIXED/Transceiver6/Interpolation 2/E4 ==
  In1 : Inport
  Data Type Conversion1 : DataTypeConversion  OutDataTypeStr=fixdt(1,18,0)  RndMeth=Floor
  Data Type Conversion12 : DataTypeConversion  OutDataTypeStr=fixdt(1,11,0)  RndMeth=Floor
  Data Type Conversion2 : DataTypeConversion  OutDataTypeStr=fixdt(1,19,0)  RndMeth=Floor
  Data Type Conversion3 : DataTypeConversion  OutDataTypeStr=fixdt(1,16,0)  RndMeth=Floor
  Data Type Conversion4 : DataTypeConversion  OutDataTypeStr=fixdt(1,18,0)  RndMeth=Floor
  Data Type Conversion5 : DataTypeConversion  OutDataTypeStr=fixdt(1,19,0)  RndMeth=Floor
  Delay3 : Delay  DelayLength=1
  Delay4 : Delay  DelayLength=1
  Delay5 : Delay  DelayLength=1
  Gain : Gain
  Gain1 : Gain  Gain=161
  Gain2 : Gain  Gain=315
  Gain3 : Gain  Gain=35
  Sum : Sum
  Sum1 : Sum
  Sum2 : Sum
  Out1 : Outport
  wires:
  Sum1/1 -> Data Type Conversion5/1
  Sum/1 -> Data Type Conversion4/1
  Gain1/1 -> Data Type Conversion1/1
  Delay3/1 -> Sum/2
  Delay4/1 -> Sum1/2
  Gain3/1 -> Data Type Conversion3/1
  Delay5/1 -> Sum2/2
  Gain/1 -> Data Type Conversion12/1
  Data Type Conversion12/1 -> Delay3/1
  Data Type Conversion1/1 -> Sum/1
  Gain2/1 -> Data Type Conversion2/1
  Data Type Conversion2/1 -> Sum1/1
  Data Type Conversion3/1 -> Sum2/1
  Data Type Conversion4/1 -> Delay4/1
  Data Type Conversion5/1 -> Delay5/1
  In1/1 -> Gain2/1, Gain3/1, Gain1/1, Gain/1
  Sum2/1 -> Out1/1

== system MIMOOO_FIXED/Transceiver6/Interpolation 2/E5 ==
  In1 : Inport
  Data Type Conversion1 : DataTypeConversion  OutDataTypeStr=fixdt(1,19,0)  RndMeth=Floor
  Data Type Conversion12 : DataTypeConversion  OutDataTypeStr=fixdt(1,18,0)  RndMeth=Floor
  Data Type Conversion2 : DataTypeConversion  OutDataTypeStr=fixdt(1,17,0)  RndMeth=Floor
  Data Type Conversion3 : DataTypeConversion  OutDataTypeStr=fixdt(1,19,0)  RndMeth=Floor
  Delay6 : Delay  DelayLength=1
  Delay7 : Delay  DelayLength=1
  Gain4 : Gain  Gain=120
  Gain5 : Gain  Gain=336
  Gain6 : Gain  Gain=56
  Sum4 : Sum
  Sum5 : Sum
  Out1 : Outport
  wires:
  Gain4/1 -> Data Type Conversion12/1
  Sum4/1 -> Data Type Conversion3/1
  Delay7/1 -> Sum5/2
  Gain6/1 -> Data Type Conversion2/1
  Delay6/1 -> Sum4/2
  Data Type Conversion12/1 -> Delay6/1
  Gain5/1 -> Data Type Conversion1/1
  Data Type Conversion1/1 -> Sum4/1
  Data Type Conversion2/1 -> Sum5/1
  Data Type Conversion3/1 -> Delay7/1
  In1/1 -> Gain6/1, Gain5/1, Gain4/1
  Sum5/1 -> Out1/1

== system MIMOOO_FIXED/Transceiver6/Interpolation 2/E6 ==
  In1 : Inport
  Data Type Conversion1 : DataTypeConversion  OutDataTypeStr=fixdt(1,20,0)  RndMeth=Floor
  Data Type Conversion2 : DataTypeConversion  OutDataTypeStr=fixdt(1,20,0)  RndMeth=Floor
  Data Type Conversion3 : DataTypeConversion  OutDataTypeStr=fixdt(1,17,0)  RndMeth=Floor
  Delay6 : Delay  DelayLength=1
  Delay7 : Delay  DelayLength=1
  Gain4 : Gain  Gain=84
  Gain5 : Gain  Gain=344
  Sum4 : Sum
  Sum5 : Sum
  Out1 : Outport
  wires:
  Delay7/1 -> Sum5/2
  Gain4/1 -> Data Type Conversion3/1
  Gain5/1 -> Data Type Conversion1/1
  Delay6/1 -> Sum4/2
  Data Type Conversion3/1 -> Sum5/1, Delay6/1
  Data Type Conversion1/1 -> Sum4/1
  Sum4/1 -> Data Type Conversion2/1
  Data Type Conversion2/1 -> Delay7/1
  In1/1 -> Gain5/1, Gain4/1
  Sum5/1 -> Out1/1

== system MIMOOO_FIXED/Transceiver6/Interpolation 2/E7 ==
  In1 : Inport
  Data Type Conversion1 : DataTypeConversion  OutDataTypeStr=fixdt(1,19,0)  RndMeth=Floor
  Data Type Conversion12 : DataTypeConversion  OutDataTypeStr=fixdt(1,17,0)  RndMeth=Floor
  Data Type Conversion2 : DataTypeConversion  OutDataTypeStr=fixdt(1,18,0)  RndMeth=Floor
  Data Type Conversion3 : DataTypeConversion  OutDataTypeStr=fixdt(1,19,0)  RndMeth=Floor
  Delay6 : Delay  DelayLength=1
  Delay7 : Delay  DelayLength=1
  Gain4 : Gain  Gain=56
  Gain5 : Gain  Gain=336
  Gain6 : Gain  Gain=120
  Sum4 : Sum
  Sum5 : Sum
  Out1 : Outport
  wires:
  Gain4/1 -> Data Type Conversion12/1
  Sum4/1 -> Data Type Conversion3/1
  Delay7/1 -> Sum5/2
  Gain6/1 -> Data Type Conversion2/1
  Delay6/1 -> Sum4/2
  Data Type Conversion12/1 -> Delay6/1
  Gain5/1 -> Data Type Conversion1/1
  Data Type Conversion1/1 -> Sum4/1
  Data Type Conversion2/1 -> Sum5/1
  Data Type Conversion3/1 -> Delay7/1
  In1/1 -> Gain6/1, Gain5/1, Gain4/1
  Sum5/1 -> Out1/1

== system MIMOOO_FIXED/Transceiver7/ADC 1/SigmaDelta ADC ==
  note: c1
  In : Inport
  Discrete Transfer Fcn : DiscreteTransferFcn  Denominator=[1 -1]
  Discrete Transfer Fcn1 : DiscreteTransferFcn  Numerator=[1 0]  Denominator=[1 -1]
  Discrete Transfer Fcn2 : DiscreteTransferFcn  Denominator=[1 -1]
  Discrete Transfer Fcn3 : DiscreteTransferFcn  Numerator=[1 0]  Denominator=[1 -1]
  Discrete Transfer Fcn4 : DiscreteTransferFcn  Denominator=[1 -1]
  Discrete Transfer Fcn5 : DiscreteTransferFcn  Numerator=[1 0]  Denominator=[1 -1]
  Sign : Signum
  Sum : Sum  Inputs=-++  InputSameDT=on  SaturateOnIntegerOverflow=on  OutDataTypeStr=Inherit: Same as first input
  Sum1 : Sum  Inputs=-+  InputSameDT=on  SaturateOnIntegerOverflow=on  OutDataTypeStr=Inherit: Same as first input
  Sum3 : Sum  Inputs=-+  InputSameDT=on  SaturateOnIntegerOverflow=on  OutDataTypeStr=Inherit: Same as first input
  Sum4 : Sum  Inputs=++++++  InputSameDT=on  SaturateOnIntegerOverflow=on  OutDataTypeStr=Inherit: Same as first input
  a : Gain  Gain=-1  SaturateOnIntegerOverflow=on  OutDataTypeStr=Inherit: Same as input  ParamDataTypeStr=Inherit: Same as input
  a1 : Gain  Gain=0.556869897897495  SaturateOnIntegerOverflow=on  OutDataTypeStr=Inherit: Same as input  ParamDataTypeStr=Inherit: Same as input
  a2 : Gain  Gain=-0.556869897925717  SaturateOnIntegerOverflow=on  OutDataTypeStr=Inherit: Same as input  ParamDataTypeStr=Inherit: Same as input
  a3 : Gain  Gain=5.57074843011795e-10  SaturateOnIntegerOverflow=on  OutDataTypeStr=Inherit: Same as input  ParamDataTypeStr=Inherit: Same as input
  a4 : Gain  Gain=-0.239860502762260  SaturateOnIntegerOverflow=on  OutDataTypeStr=Inherit: Same as input  ParamDataTypeStr=Inherit: Same as input
  a5 : Gain  Gain=-0.0411685762497780  SaturateOnIntegerOverflow=on  OutDataTypeStr=Inherit: Same as input  ParamDataTypeStr=Inherit: Same as input
  a6 : Gain  Gain=0.0229325751731016  SaturateOnIntegerOverflow=on  OutDataTypeStr=Inherit: Same as input  ParamDataTypeStr=Inherit: Same as input
  gc1 : Gain  Gain=2.00000000000000  SaturateOnIntegerOverflow=on  OutDataTypeStr=Inherit: Same as input  ParamDataTypeStr=Inherit: Same as input
  gc2 : Gain  Gain=2.07602752770857  SaturateOnIntegerOverflow=on  OutDataTypeStr=Inherit: Same as input  ParamDataTypeStr=Inherit: Same as input
  gc3 : Gain  Gain=1.92397247229143  SaturateOnIntegerOverflow=on  OutDataTypeStr=Inherit: Same as input  ParamDataTypeStr=Inherit: Same as input
  Out : Outport
  wires:
  gc1/1 -> Sum/1
  a5/1 -> Sum4/2
  Discrete Transfer Fcn2/1 -> Discrete Transfer Fcn3/1, a3/1
  Sum4/1 -> Sign/1
  Sum1/1 -> Discrete Transfer Fcn2/1
  Sum/1 -> Discrete Transfer Fcn/1
  a1/1 -> Sum4/6
  gc2/1 -> Sum1/1
  a/1 -> Sum/3
  Discrete Transfer Fcn3/1 -> a4/1, Sum3/2, gc2/1
  Discrete Transfer Fcn5/1 -> a6/1, gc3/1
  Discrete Transfer Fcn1/1 -> a2/1, gc1/1, Sum1/2
  In/1 -> Sum/2
  Sign/1 -> Out/1, a/1
  gc3/1 -> Sum3/1
  a3/1 -> Sum4/4
  a4/1 -> Sum4/3
  a2/1 -> Sum4/5
  Discrete Transfer Fcn/1 -> Discrete Transfer Fcn1/1, a1/1
  Sum3/1 -> Discrete Transfer Fcn4/1
  Discrete Transfer Fcn4/1 -> Discrete Transfer Fcn5/1, a5/1
  a6/1 -> Sum4/1

== system MIMOOO_FIXED/Transceiver7/Interpolation 1/Half_band ==
  Input : Inport
  Add2 : Sum
  Delay11 : Delay  DelayLength=1
  E0(Z) : Subsystem
  E1(Z) : Subsystem
  Upsample 1 : dspsigops/Upsample  N=2  phase=0  RateOptions=Allow multirate processing  ic=0  mode=Unused parameter value
  Upsample 2 : dspsigops/Upsample  N=2  phase=0  RateOptions=Allow multirate processing  ic=0  mode=Unused parameter value
  Out1 : Outport
  wires:
  Upsample 2/1 -> Delay11/1
  Upsample 1/1 -> Add2/1
  E1(Z)/1(Output) -> Upsample 2/1
  Delay11/1 -> Add2/2
  E0(Z)/1(Out1) -> Upsample 1/1
  Add2/1 -> Out1/1
  Input/1 -> E0(Z)/1(Input), E1(Z)/1(Input1)

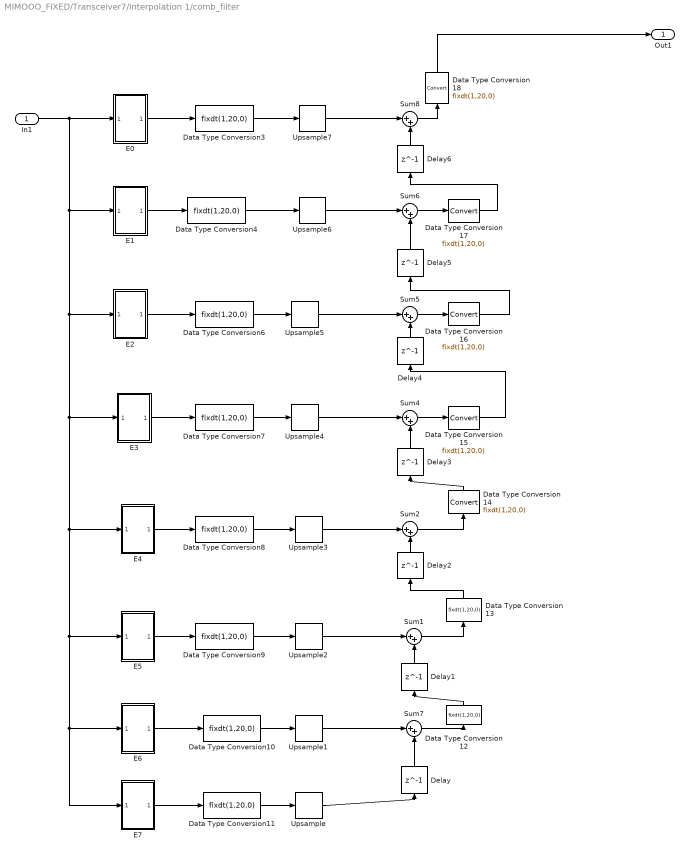
== system MIMOOO_FIXED/Transceiver7/Interpolation 1/comb_filter ==
  In1 : Inport
  Data Type Conversion{3..4,6..18} (15 alike) : DataTypeConversion  OutDataTypeStr=fixdt(1,20,0)  RndMeth=Floor
  Delay{,1..6} (7 alike) : Delay  DelayLength=1
  E0 : Subsystem
  E1 : Subsystem
  E2 : Subsystem
  E3 : Subsystem
  E4 : Subsystem
  E5 : Subsystem
  E6 : Subsystem
  E7 : Subsystem
  Sum{1..2,4..8} (7 alike) : Sum  Inputs=|++
  Upsample{,1..7} (8 alike) : dspsigops/Upsample  N=8  phase=0  RateOptions=Allow multirate processing  ic=0  mode=Unused parameter value
  Out1 : Outport
  wires:
  Upsample7/1 -> Sum8/1
  E4/1(Out1) -> Data Type Conversion8/1
  Data Type Conversion4/1 -> Upsample6/1
  E6/1(Out1) -> Data Type Conversion10/1
  Delay4/1 -> Sum5/2
  Data Type Conversion13/1 -> Delay2/1
  Delay5/1 -> Sum6/2
  Data Type Conversion9/1 -> Upsample2/1
  Sum8/1 -> Data Type Conversion18/1
  Data Type Conversion3/1 -> Upsample7/1
  Sum6/1 -> Data Type Conversion17/1
  Data Type Conversion15/1 -> Delay4/1
  Data Type Conversion14/1 -> Delay3/1
  Data Type Conversion16/1 -> Delay5/1
  E2/1(Out1) -> Data Type Conversion6/1
  In1/1 -> E0/1(In1), E7/1(In1), E6/1(In1), E5/1(In1), E4/1(In1), E3/1(In1), E2/1(In1), E1/1(In1)
  Delay2/1 -> Sum2/2
  Data Type Conversion17/1 -> Delay6/1
  Sum7/1 -> Data Type Conversion12/1
  Data Type Conversion6/1 -> Upsample5/1
  Sum2/1 -> Data Type Conversion14/1
  Data Type Conversion10/1 -> Upsample1/1
  Upsample/1 -> Delay/1
  Upsample6/1 -> Sum6/1
  E5/1(Out1) -> Data Type Conversion9/1
  Data Type Conversion8/1 -> Upsample3/1
  Data Type Conversion7/1 -> Upsample4/1
  Delay1/1 -> Sum1/2
  Sum5/1 -> Data Type Conversion16/1
  Delay/1 -> Sum7/2
  Upsample3/1 -> Sum2/1
  Data Type Conversion11/1 -> Upsample/1
  Upsample4/1 -> Sum4/1
  E7/1(Out1) -> Data Type Conversion11/1
  Sum1/1 -> Data Type Conversion13/1
  Delay3/1 -> Sum4/2
  E3/1(Out1) -> Data Type Conversion7/1
  Data Type Conversion12/1 -> Delay1/1
  Sum4/1 -> Data Type Conversion15/1
  Upsample2/1 -> Sum1/1
  Upsample5/1 -> Sum5/1
  Upsample1/1 -> Sum7/1
  E1/1(Out1) -> Data Type Conversion4/1
  Delay6/1 -> Sum8/2
  Data Type Conversion18/1 -> Out1/1
  E0/1(Out1) -> Data Type Conversion3/1

== system MIMOOO_FIXED/Transceiver7/Interpolation 2/E0 ==
  In1 : Inport
  Data Type Conversion1 : DataTypeConversion  OutDataTypeStr=fixdt(1,19,0)  RndMeth=Floor
  Data Type Conversion2 : DataTypeConversion  OutDataTypeStr=fixdt(1,18,0)  RndMeth=Floor
  Data Type Conversion3 : DataTypeConversion  OutDataTypeStr=fixdt(1,11,0)  RndMeth=Floor
  Data Type Conversion4 : DataTypeConversion  OutDataTypeStr=fixdt(1,20,0)  RndMeth=Floor
  Data Type Conversion5 : DataTypeConversion  OutDataTypeStr=fixdt(1,20,0)  RndMeth=Floor
  Data Type Conversion7 : DataTypeConversion  OutDataTypeStr=fixdt(1,16,0)  RndMeth=Floor
  Delay3 : Delay  DelayLength=1
  Delay4 : Delay  DelayLength=1
  Delay5 : Delay  DelayLength=1
  Gain : Gain  Gain=35
  Gain1 : Gain  Gain=315
  Gain2 : Gain  Gain=161
  Gain3 : Gain
  Sum : Sum
  Sum1 : Sum
  Sum2 : Sum
  Out1 : Outport
  wires:
  Sum1/1 -> Data Type Conversion5/1
  Delay3/1 -> Sum/2
  Delay5/1 -> Sum2/2
  Data Type Conversion7/1 -> Delay3/1
  Gain/1 -> Data Type Conversion7/1
  Gain1/1 -> Data Type Conversion1/1
  Data Type Conversion1/1 -> Sum/1
  Gain2/1 -> Data Type Conversion2/1
  Data Type Conversion3/1 -> Sum2/1
  Gain3/1 -> Data Type Conversion3/1
  Sum/1 -> Data Type Conversion4/1
  Data Type Conversion4/1 -> Delay4/1
  Data Type Conversion2/1 -> Sum1/1
  Delay4/1 -> Sum1/2
  Data Type Conversion5/1 -> Delay5/1
  In1/1 -> Gain2/1, Gain3/1, Gain1/1, Gain/1
  Sum2/1 -> Out1/1

== system MIMOOO_FIXED/Transceiver7/Interpolation 2/E0(Z) ==
  Input : Inport
  Data Type Conversion5 : DataTypeConversion  OutDataTypeStr=fixdt(1,23,0)  RndMeth=Floor
  Delay : Delay  DelayLength=5
  Gain : Gain  Gain=256
  Out1 : Outport
  wires:
  Input/1 -> Gain/1
  Delay/1 -> Out1/1
  Gain/1 -> Data Type Conversion5/1
  Data Type Conversion5/1 -> Delay/1

== system MIMOOO_FIXED/Transceiver7/Interpolation 2/E1 ==
  In1 : Inport
  Data Type Conversion1 : DataTypeConversion  OutDataTypeStr=fixdt(1,19,0)  RndMeth=Floor
  Data Type Conversion2 : DataTypeConversion  OutDataTypeStr=fixdt(1,19,0)  RndMeth=Floor
  Data Type Conversion3 : DataTypeConversion  OutDataTypeStr=fixdt(1,13,0)  RndMeth=Floor
  Data Type Conversion4 : DataTypeConversion  OutDataTypeStr=fixdt(1,19,0)  RndMeth=Floor
  Data Type Conversion5 : DataTypeConversion  OutDataTypeStr=fixdt(1,20,0)  RndMeth=Floor
  Data Type Conversion7 : DataTypeConversion  OutDataTypeStr=fixdt(1,15,0)  RndMeth=Floor
  Delay3 : Delay  DelayLength=1
  Delay4 : Delay  DelayLength=1
  Delay5 : Delay  DelayLength=1
  Gain : Gain  Gain=20
  Gain1 : Gain  Gain=284
  Gain2 : Gain  Gain=204
  Gain3 : Gain  Gain=4
  Sum : Sum
  Sum1 : Sum
  Sum2 : Sum
  Out1 : Outport
  wires:
  Sum/1 -> Data Type Conversion4/1
  Delay3/1 -> Sum/2
  Delay4/1 -> Sum1/2
  Delay5/1 -> Sum2/2
  Gain/1 -> Data Type Conversion7/1
  Data Type Conversion7/1 -> Delay3/1
  Gain1/1 -> Data Type Conversion1/1
  Data Type Conversion1/1 -> Sum/1
  Gain2/1 -> Data Type Conversion2/1
  Data Type Conversion2/1 -> Sum1/1
  Gain3/1 -> Data Type Conversion3/1
  Data Type Conversion3/1 -> Sum2/1
  Data Type Conversion4/1 -> Delay4/1
  Sum1/1 -> Data Type Conversion5/1
  Data Type Conversion5/1 -> Delay5/1
  In1/1 -> Gain2/1, Gain3/1, Gain1/1, Gain/1
  Sum2/1 -> Out1/1
